simulink model "Simulate"  (R2015a)
settings: Solver=ode45  StartTime=0.0  StopTime=10.0  RelTol=1e-3
settings Model: Creator=Yash  LastModifiedBy=Yash

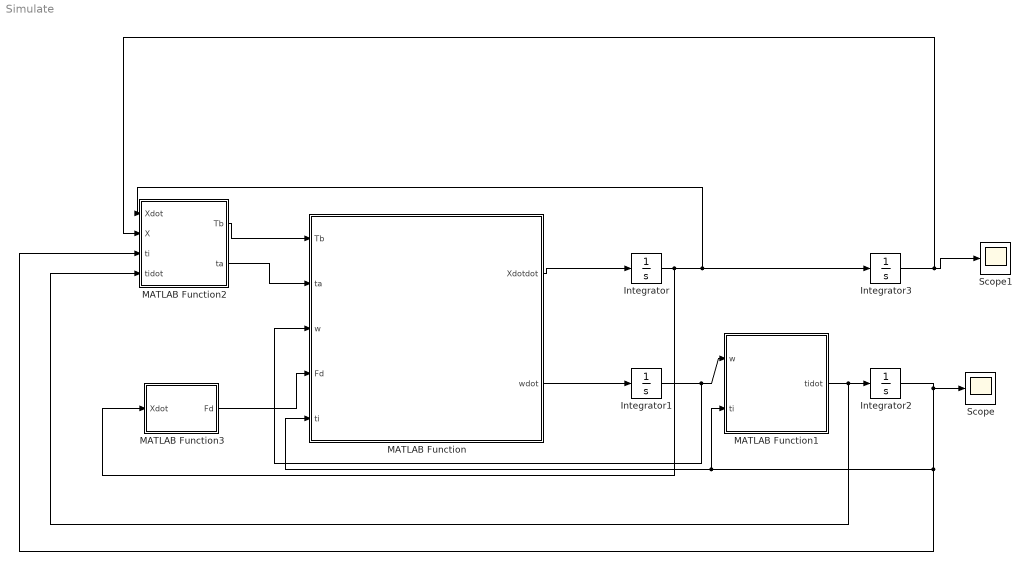
== system Simulate ==
  Integrator : Integrator  InitialCondition=[0;0;0]
  Integrator1 : Integrator  InitialCondition=[0;0;0]
  Integrator2 : Integrator  InitialCondition=[pi/18;pi/18;pi/18]
  Integrator3 : Integrator  InitialCondition=[0;0;1]
  MATLAB Function : MATLAB Function  TreatAsAtomicUnit=on
  MATLAB Function1 : MATLAB Function  TreatAsAtomicUnit=on
  MATLAB Function2 : MATLAB Function  TreatAsAtomicUnit=on
  MATLAB Function3 : MATLAB Function  TreatAsAtomicUnit=on
  Scope : Scope
  Scope1 : Scope
  wires:
  MATLAB Function/1(Xdotdot) -> Integrator/1
  MATLAB Function/2(wdot) -> Integrator1/1
  MATLAB Function2/1(Tb) -> MATLAB Function/1(Tb)
  Integrator/1 -> MATLAB Function3/1(Xdot), MATLAB Function2/1(Xdot), Integrator3/1
  MATLAB Function3/1(Fd) -> MATLAB Function/4(Fd)
  Integrator1/1 -> MATLAB Function/3(w), MATLAB Function1/1(w)
  MATLAB Function2/2(ta) -> MATLAB Function/2(ta)
  Integrator3/1 -> MATLAB Function2/2(X), Scope1/1
  MATLAB Function1/1(tidot) -> MATLAB Function2/4(tidot), Integrator2/1
  Integrator2/1 -> MATLAB Function2/3(ti), MATLAB Function1/2(ti), MATLAB Function/5(ti), Scope/1

== matlab function Simulate/MATLAB Function1 ==
  data: w input; tidot output; ti input
function tidot = fcn(w,ti)

tita=ti(1);
phi=ti(2);

Z=[1 0 -sin(tita);
    0 cos(phi) cos(tita)*sin(phi);
    0 -sin(phi) cos(tita)*cos(phi)];

tidot= Z\w;

== matlab function Simulate/MATLAB Function ==
  data: Tb input; ta input; w input; Fd input; Xdotdot output; wdot output; ti input
function [Xdotdot,wdot]= fcn(Tb,ta,w,Fd,ti)

phi=ti(1);
tita=ti(2);
xi=ti(3);
Ixx=4.856e-3;
Iyy=4.856e-3;
Izz=8.801e-3;
g=9.81;
m=0.468;

R= [cos(phi)*cos(xi)-cos(tita)*son(phi)*sin(xi) -cos(xi)*sin(phi)-cos(phi)*cos(tita)*sin(xi) sin(tita)*sin(xi);
    cos(tita)*cos(xi)*sin(phi) cos(phi)*cos(tita)*cos(xi)-sin(phi)*sin(xi) -cos(xi)*sin(tita);
    sin(phi)*sin(tita) cos(phi)*sin(tita) cos(tita)];

I= [Ixx 0 0;
    0 Iyy 0;
    0 0 Izz];


wdot= I\(ta-wcrossI*w);

Xdotdot= [0;0;-g] + R*Tb/m + Fd/m;

== matlab function Simulate/MATLAB Function2 ==
  data: Xdot input; Tb output; ta output; X input; ti input; tidot input
function [Tb,ta]= fcn(Xdot,X,ti,tidot)


l=0.225;
k=2.98e-6;
b=1.14e-7;
phi=ti(1);
tita=ti(2);
xi=ti(3);
zdot=Xdot(3);
z=X(1);
g=9.81;
phidot=tidot(1);
titadot=tidot(2);
xidot=tidot(3);
Kzd=2.5;
Kzp=1.5;
Kd=1.75;
Kp=6;




T = (g + Kzd(zddot-zdot) + Kzp(zd-z))*m/(cos(phi)*cos(tita));
tap = (Kd(phiddot-phidot) + Kp(phid-phi))*Ixx;
tat = (Kd(titaddot-titadot) + Kp(titad-tita))*Iyy;
tax = (Kd(xiddot-xidot) + Kp(xid-xi))*Izz;



w1 = T/(4*k) -tat/(2*k*l) -tax/(4*b);
w2 = T/(4*k) -tap/(2*k*l) +tax/(4*b);
w3 = T/(4*k) +tat/(2*k*l) -tax/(4*b);
w4 = T/(4*k) +tap/(2*k*l) +tax/(4*b);

Tb=[0;
    0;
    power(w1,2)+power(w2,2)+power(w3,2)+power(w4,2)];

ta= [l*k*(power(w1,2)-power(w3,2));
     l*k*(power(w2,2)-power(w4,2));
     b*(power(w1,2)-power(w2,2)+power(w3,2)-power(w4,2))];

== matlab function Simulate/MATLAB Function3 ==
  data: Xdot input; Fd output
function Fd = fcn(Xdot)
xdot= Xdot(1);
ydot= Xdot(2);
zdot= Xdot(3);
kd=0.25;

Fd=[-kd*xdot;
    -kd*ydot;
    -kd*zdot];
